simulink model "Motor_Model"  (R2020b)
settings: Solver=VariableStepAuto  StartTime=0.0  StopTime=5  RelTol=1e-3
libraries: fl_lib x114, ee_lib x34, nesl_utility x20
(part 1 of 2)
settings Model: SimulationMode=accelerator  Creator=rubse  LastModifiedBy=rubse

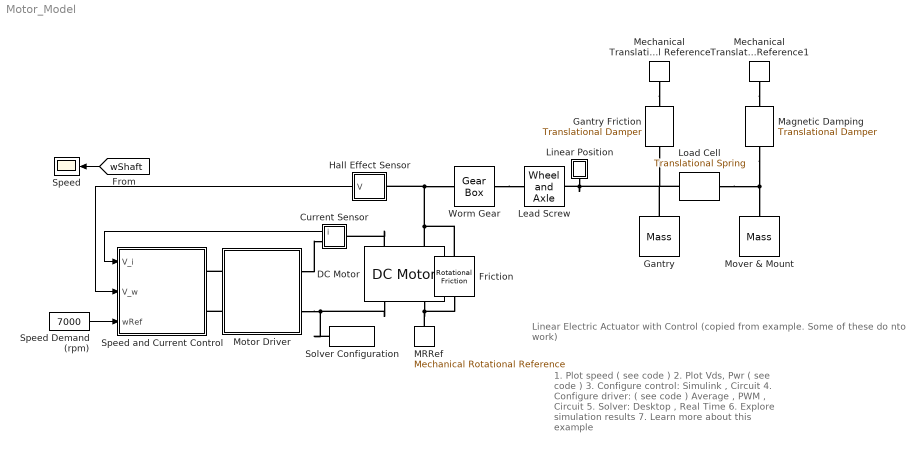
== system Motor_Model ==
  note: Linear Electric Actuator with Control
      | (copied from example. Some of these do nto work)
  note: 1. Plot speed ( see code )
      | 2. Plot Vds, Pwr ( see code )
      | 3. Configure control: Simulink , Circuit
      | 4. Configure driver: ( see code )
      | Average , PWM , Circuit
      | 5. Solver: Desktop , Real Time
      | 6. Explore simulation results
      | 7. Learn more about this example
  Current Sensor : Subsystem
  DC Motor : ee_lib/Electromechanical/Brushed Motors/DC Motor  field_option=ee.enum.field_option.pm  Rf=100 Ohm  Lf=1 H  Laf=0.15 H  If0=0 A  parameterization=ee.enum.dcparam_option.circuit_param  Ra=0.0787 Ohm  La=0.121e-3 H  emf_or_torque=ee.enum.emf_or_torque.ki  Kv=0.0637 V/rpm  Ki=32.3e-3 N*m/A  T_stall=2.4e-4 N*m  w_max=1.91e+4 rpm  w_rated=1.5e+4 rpm  P_rated=0.08 W  V_rated=1.5 V  J=107 g*cm^2  lam_param=ee.enum.lam_param.damping  lam=1e-08 N*m/(rad/s)  i_noload=0 A  V_i_noload=1.5 V  speed0=0 rpm  enable_fault_armature=ee.enum.faults.faultEnable.no  rev_faulted=1 / 3  G_faulted_armature=1e-5 S  fault_trigger_armature=ee.enum.faults.faultTrigger.temporal  t_fault_armature=1 s  max_permissible_current_armature=inf A  t_fail_on_current_armature=1 s  enable_fault_field=ee.enum.faults.faultEnable.no  G_faulted_field=1e-5 S  fault_trigger_field=ee.enum.faults.faultTrigger.temporal  t_fault_field=1 s  max_permissible_current_field=inf A  t_fail_on_current_field=1 s  fault_action=ee.enum.faults.faultAction.none  alpha=3.93e-3 1/K  Tmeas=25 degC  thermal_mass=100 J/K  initial_temperature=25 degC
      settings: SourceProductName=Electrical
  Friction : fl_lib/Mechanical/Rotational Elements/Rotational Friction  brkwy_trq=0.022 N*m  brkwy_vel=0.03347 rad/s  Col_trq=0.022 N*m  visc_coef=0 N*m/(rad/s)  w_specify=off  w_priority=High  w=0 rad/s  w_nominal_specify=off  w_nominal_unit=rad/s  w_nominal_value=1  t_specify=off  t_priority=High  t=0 N*m  t_nominal_specify=off  t_nominal_unit=N*m  t_nominal_value=1
      settings: SourceProductName=Foundation Library
  Gantry : fl_lib/Mechanical/Translational Elements/Mass  mass=5 kg  num_ports=foundation.enum.numPorts2.one  v_specify=off  v_priority=High  v=0 m/s  v_nominal_specify=off  v_nominal_unit=m/s  v_nominal_value=1  f_specify=off  f_priority=None  f=0 N  f_nominal_specify=off  f_nominal_unit=N  f_nominal_value=1
  Gantry Friction : fl_lib/Mechanical/Translational Elements/Translational Damper  D=0.09 N/(m/s)  v_specify=off  v_priority=None  v=0 m/s  v_nominal_specify=off  v_nominal_unit=m/s  v_nominal_value=1  f_specify=off  f_priority=None  f=0 N  f_nominal_specify=off  f_nominal_unit=N  f_nominal_value=1
  Hall Effect Sensor : Subsystem
  Lead Screw : fl_lib/Mechanical/Mechanisms/Wheel and Axle  R=0.05 m  or=1  t_specify=off  t_priority=High  t=0 N*m  t_nominal_specify=off  t_nominal_unit=N*m  t_nominal_value=1  f_specify=off  f_priority=High  f=0 N  f_nominal_specify=off  f_nominal_unit=N  f_nominal_value=1
      settings: SourceProductName=Foundation Library
  Linear Position : Subsystem
      mask Display: disp('S');
  Load Cell : fl_lib/Mechanical/Translational Elements/Translational Spring  spr_rate=670000 N/m  v_specify=off  v_priority=None  v=0 m/s  v_nominal_specify=off  v_nominal_unit=m/s  v_nominal_value=1  f_specify=off  f_priority=None  f=0 N  f_nominal_specify=off  f_nominal_unit=N  f_nominal_value=1  x_specify=off  x_priority=High  x=0 m  x_nominal_specify=off  x_nominal_unit=m  x_nominal_value=1
  MRRef : fl_lib/Mechanical/Rotational Elements/Mechanical Rotational Reference
      settings: SourceProductName=Foundation Library
  Magnetic Damping : fl_lib/Mechanical/Translational Elements/Translational Damper  D=49.05 N/(m/s)  v_specify=off  v_priority=None  v=0 m/s  v_nominal_specify=off  v_nominal_unit=m/s  v_nominal_value=1  f_specify=off  f_priority=None  f=0 N  f_nominal_specify=off  f_nominal_unit=N  f_nominal_value=1
  Mechanical Translational Reference : fl_lib/Mechanical/Translational Elements/Mechanical Translational Reference
  Mechanical Translational Reference1 : fl_lib/Mechanical/Translational Elements/Mechanical Translational Reference
  Motor Driver : Subsystem  Variant=on  VariantControlMode=label  LabelModeActiveChoice=Circuit
      settings: AttributesFormatString=%<ActiveVariant>
      mask Display:
      | if(strcmp(get_param(gcb,'ActiveVariant'),'Circuit'))
      |     temp_imagename = 'ee_motor_linact_control_drive_circuit.jpg';
      | elseif(strcmp(get_param([gcb '/Abstract/Controlled PWM Voltage'],'pwm_or_av'),'1'))
      |     temp_imagename = 'ee_motor_linact_control_drive_abstract_pwm.jpg';
      | else
      |     temp_imagename = 'ee_motor_linact_control_drive_abstract_continuous.jpg';
      | end
      | 
      | image(imread(temp_imagename));
  Mover & Mount : fl_lib/Mechanical/Translational Elements/Mass  mass=2.03 kg  num_ports=foundation.enum.numPorts2.one  v_specify=off  v_priority=High  v=0 m/s  v_nominal_specify=off  v_nominal_unit=m/s  v_nominal_value=1  f_specify=off  f_priority=None  f=0 N  f_nominal_specify=off  f_nominal_unit=N  f_nominal_value=1
  Solver Configuration : nesl_utility/Solver Configuration  PhysicalDomain=network_engine_domain  SubClassName=solver  LeftPortType=input  RightPortType=generic  Tones=[]  Harmonics=[]  SimulateNoise=off  Profile=off  UseLocalSampling=off  EnableSwitchedLinearOptims=on  FrequencyDomain=off  UseCCode=off  RelTol=0.001  AbsTol=1e-06  MinStep=1e-09  ToWorkspace=off  RevertToSquareIcSolve=off  NumHomotopyIterations=100  PhasorMode=off  PhasorModeNumHarmonics=1  DoDC=off  ResidualTolerance=1e-9  UseLocalSolver=off  LocalSolverChoice=NE_BACKWARD_EULER_ADVANCER  LocalSolverSampleTime=0.0001  DoFixedCost=off  MaxNonlinIter=3  MaxModeIter=2  ComputeImpulses=off  ImpulseIterations=2  LinearAlgebra=auto  EquationFormulation=NE_TIME_EF  DelaysMemoryBudget=1024  AutomaticFiltering=on  FilteringTimeConstant=0.001  PartitionStorageMethod=AS_NEEDED  PartitionMemoryBudget=1024  PartitionMethod=FAST
      settings: SourceProductName=Utilities
  Speed : Scope
  Speed Demand (rpm) : Constant  Value=7000
  Speed and Current Control : Subsystem  Variant=on  VariantControlMode=label  LabelModeActiveChoice=Simulink
      settings: AttributesFormatString=%<ActiveVariant>
      mask Display:
      | blk = find_system(gcbh, 'SearchDepth', 1, 'Parent', gcb, 'VariantObject', get_param(gcb,'activevariant'));
      | eval(get_param(blk, 'MaskDisplay'));
  Worm Gear : fl_lib/Mechanical/Mechanisms/Gear Box  ratio=12  t_in_specify=off  t_in_priority=High  t_in=0 N*m  t_in_nominal_specify=off  t_in_nominal_unit=N*m  t_in_nominal_value=1  t_out_specify=off  t_out_priority=High  t_out=0 N*m  t_out_nominal_specify=off  t_out_nominal_unit=N*m  t_out_nominal_value=1
      settings: SourceProductName=Foundation Library
  wires:
  Speed Demand (rpm)/1 -> Speed and Current Control/3(wRef)
  Current Sensor/1(i) -> Speed and Current Control/1(V_i)
  Hall Effect Sensor/1(V) -> Speed and Current Control/2(V_w)
  [wShaft] -> Speed/1
  connections:
  DC Motor/RConn2 -- MRRef/LConn1 -- Friction/RConn1
  DC Motor/LConn2 -- Worm Gear/LConn1 -- Hall Effect Sensor/LConn1 -- Friction/LConn1
  Linear Position/LConn1 -- Load Cell/LConn1 -- Gantry/LConn1 -- Gantry Friction/RConn1 -- Lead Screw/RConn1
  Solver Configuration/RConn1 -- DC Motor/RConn1 -- Motor Driver/RConn2
  Motor Driver/LConn2 -- Speed and Current Control/RConn2
  Motor Driver/LConn1 -- Speed and Current Control/RConn1
  DC Motor/LConn1 -- Current Sensor/LConn1
  Motor Driver/RConn1 -- Current Sensor/RConn1
  Worm Gear/RConn1 -- Lead Screw/LConn1
  Mechanical Translational Reference/LConn1 -- Gantry Friction/LConn1
  Load Cell/RConn1 -- Mover & Mount/LConn1 -- Magnetic Damping/RConn1
  Mechanical Translational Reference1/LConn1 -- Magnetic Damping/LConn1

== system Motor_Model/Current Sensor ==
  2kHz Lowpass Filter : TransferFcn  Denominator=[1/(2*pi*1000) 1]
  Current Sensor : fl_lib/Electrical/Electrical Sensors/Current Sensor
      settings: SourceProductName=Foundation Library
  Motor Current : Scope
  PS-Simulink Converter 2 : nesl_utility/PS-Simulink Converter  PhysicalDomain=network_engine_domain  SubClassName=ps_output  LeftPortType=input  RightPortType=output  PseudoPeriodic=off  Frequencies=[]  Unit=A  AffineConversion=off
      settings: SourceProductName=Utilities
  + : PMIOPort  Side=Right
  - : PMIOPort  Port=2  Side=Left
  i : Outport  VectorParamsAs1DForOutWhenUnconnected=off
  wires:
  PS-Simulink Converter 2/1 -> 2kHz Lowpass Filter/1, Motor Current/1  "Current (A)"
  2kHz Lowpass Filter/1 -> i/1
  connections:
  +/RConn1 -- Current Sensor/LConn1
  -/RConn1 -- Current Sensor/RConn2
  Current Sensor/RConn1 -- PS-Simulink Converter 2/LConn1

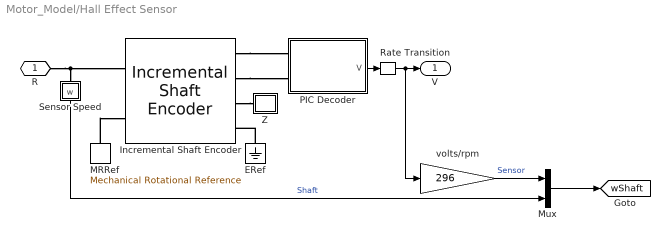
== system Motor_Model/Hall Effect Sensor ==
  ERef : fl_lib/Electrical/Electrical Elements/Electrical Reference
      settings: SourceProductName=Foundation Library
  Incremental Shaft Encoder : ee_lib/Sensors & Transducers/Incremental Shaft Encoder  NPulse=2  Vm=5 V  angle0=-1 deg
      settings: SourceProductName=Electrical  InternalSimscapePortConfiguration="{\"Bottom\":[],\"Left\":[{\"id\":\"R\",\"label\":\"R\",\"type\":\"foundation.mechanical.rotational.rotational\"},{\"id\":\"C\",\"label\":\"C\",\"type\":\"foundation.mechanical.rotational.rotational\"}],\"Right\":[{\"id\":\"A\",\"label\":\"A\",\"type\":\"foundation.electrical.electrical\"},{\"id\":\"B\",\"label\":\"B\",\"type\":\"foundation.electrical.electrical\"},{\"id\":\"Z\",\"label\":\"Z\",\"type\":\"foundation.electrical.electrical\"},{\"id\":\"GND\",\"label\":\"REF\",\"type\":\"foundation.electrical.electrical\"}],\"Top\":[]}"
  MRRef : fl_lib/Mechanical/Rotational Elements/Mechanical Rotational Reference
      settings: SourceProductName=Foundation Library
  Mux : Mux  Inputs=2
  PIC Decoder : Subsystem
  Rate Transition : RateTransition
  Sensor Speed : Subsystem
      mask Display: disp('w')
  Z : Subsystem
  volts/rpm : Gain  Gain=296
  R : PMIOPort  Side=Left
  V : Outport  VectorParamsAs1DForOutWhenUnconnected=off
  tag scope: wShaft=global
  wires:
  PIC Decoder/1(V) -> Rate Transition/1
  Rate Transition/1 -> V/1, volts/rpm/1
  Mux/1 -> [wShaft]
  volts/rpm/1 -> Mux/1  "Sensor"
  Sensor Speed/1(w) -> Mux/2  "Shaft"
  connections:
  MRRef/LConn1 -- Incremental Shaft Encoder/LConn2
  R/RConn1 -- Incremental Shaft Encoder/LConn1 -- Sensor Speed/LConn1
  ERef/LConn1 -- Incremental Shaft Encoder/RConn4
  Incremental Shaft Encoder/RConn3 -- Z/LConn1
  Incremental Shaft Encoder/RConn1 -- PIC Decoder/LConn1
  Incremental Shaft Encoder/RConn2 -- PIC Decoder/LConn2

== system Motor_Model/Linear Position ==
  Linear Position (mm) : Scope
  Linear Speed (mm/s) : Scope
  MTRef : fl_lib/Mechanical/Translational Elements/Mechanical Translational Reference
      settings: SourceProductName=Foundation Library
  Motion Sensor : fl_lib/Mechanical/Mechanical Sensors/Ideal Translational Motion Sensor  offset=0 m
      settings: SourceProductName=Foundation Library
  PS-Simulink Converter 1 : nesl_utility/PS-Simulink Converter  PhysicalDomain=network_engine_domain  SubClassName=ps_output  LeftPortType=input  RightPortType=output  PseudoPeriodic=off  Frequencies=[]  Unit=mm/s  AffineConversion=off
      settings: SourceProductName=Utilities
  PS-Simulink Converter 3 : nesl_utility/PS-Simulink Converter  PhysicalDomain=network_engine_domain  SubClassName=ps_output  LeftPortType=input  RightPortType=output  PseudoPeriodic=off  Frequencies=[]  Unit=mm  AffineConversion=off
      settings: SourceProductName=Utilities
  P : PMIOPort  Side=Left
  wires:
  PS-Simulink Converter 3/1 -> Linear Position (mm)/1
  PS-Simulink Converter 1/1 -> Linear Speed (mm/s)/1
  connections:
  Motion Sensor/RConn1 -- MTRef/LConn1
  Motion Sensor/RConn3 -- PS-Simulink Converter 3/LConn1
  P/RConn1 -- Motion Sensor/LConn1
  Motion Sensor/RConn2 -- PS-Simulink Converter 1/LConn1

== system Motor_Model/Motor Driver ==
  Abstract : Subsystem  Tag=PublishSubsystem  VariantControl=Abstract
  Circuit : Subsystem  Tag=PublishSubsystem  VariantControl=Circuit
  + : PMIOPort  Side=Right
  - : PMIOPort  Port=2  Side=Right
  +ref : PMIOPort  Port=3  Side=Left
  REV : PMIOPort  Port=4  Side=Left

== system Motor_Model/Speed and Current Control ==
  V_i : Inport
  V_w : Inport  Port=2
  wRef : Inport  Port=3
  Circuit : Subsystem  VariantControl=Circuit
      mask Display: image(imread('ee_motor_linact_control_ctrl_circuit.jpg'));
  Simulink : Subsystem  VariantControl=Simulink
      mask Display: image('ee_motor_linact_control_ctrl_simulink.jpg');
  Vr : PMIOPort  Side=Right
  REV : PMIOPort  Port=2  Side=Right

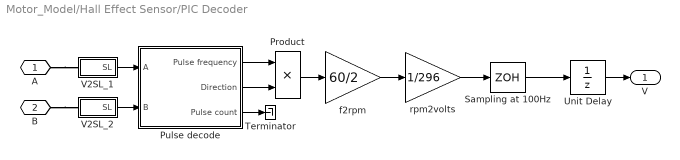
== system Motor_Model/Hall Effect Sensor/PIC Decoder ==
  Product : Product  RndMeth=Zero
  Pulse decode : Subsystem
  Sampling at 100Hz : ZeroOrderHold  SampleTime=0.01
  Terminator : Terminator
  Unit Delay : UnitDelay  SampleTime=0.01  HasFrameUpgradeWarning=on
  V2SL_1 : Subsystem
  V2SL_2 : Subsystem
  f2rpm : Gain  Gain=60/2
  rpm2volts : Gain  Gain=1/296
  A : PMIOPort  Side=Left
  B : PMIOPort  Port=2  Side=Left
  V : Outport  VectorParamsAs1DForOutWhenUnconnected=off
  wires:
  Product/1 -> f2rpm/1
  Pulse decode/2(Direction) -> Product/2
  Pulse decode/1(Pulse frequency) -> Product/1
  Pulse decode/3(Pulse count) -> Terminator/1
  f2rpm/1 -> rpm2volts/1
  rpm2volts/1 -> Sampling at 100Hz/1
  V2SL_1/1(SL) -> Pulse decode/1(A)
  V2SL_2/1(SL) -> Pulse decode/2(B)
  Sampling at 100Hz/1 -> Unit Delay/1
  Unit Delay/1 -> V/1
  connections:
  A/RConn1 -- V2SL_1/LConn1
  B/RConn1 -- V2SL_2/LConn1

== system Motor_Model/Hall Effect Sensor/Sensor Speed ==
  MRRef5 : fl_lib/Mechanical/Rotational Elements/Mechanical Rotational Reference
      settings: SourceProductName=Foundation Library
  Motion Sensor : fl_lib/Mechanical/Mechanical Sensors/Ideal Rotational Motion Sensor  wrap_angle=simscape.enum.onoff.off  offset=0 rad
      settings: SourceProductName=Foundation Library
  PS-Simulink Converter 2 : nesl_utility/PS-Simulink Converter  PhysicalDomain=network_engine_domain  SubClassName=ps_output  LeftPortType=input  RightPortType=output  PseudoPeriodic=off  Frequencies=[]  Unit=rpm  AffineConversion=off
      settings: SourceProductName=Utilities
  R : PMIOPort  Side=Left
  w : Outport  VectorParamsAs1DForOutWhenUnconnected=off
  wires:
  PS-Simulink Converter 2/1 -> w/1
  connections:
  Motion Sensor/RConn2 -- PS-Simulink Converter 2/LConn1
  R/RConn1 -- Motion Sensor/LConn1
  MRRef5/LConn1 -- Motion Sensor/RConn1

== system Motor_Model/Hall Effect Sensor/Z ==
  ERef : fl_lib/Electrical/Electrical Elements/Electrical Reference
      settings: SourceProductName=Foundation Library
  PS-Simulink Converter 2 : nesl_utility/PS-Simulink Converter  PhysicalDomain=network_engine_domain  SubClassName=ps_output  LeftPortType=input  RightPortType=output  PseudoPeriodic=off  Frequencies=[]  Unit=V  AffineConversion=off
      settings: SourceProductName=Utilities
  Voltage Sensor : fl_lib/Electrical/Electrical Sensors/Voltage Sensor
      settings: SourceProductName=Foundation Library
  Vz : Scope
  u : PMIOPort  Side=Left
  wires:
  PS-Simulink Converter 2/1 -> Vz/1
  connections:
  Voltage Sensor/RConn2 -- ERef/LConn1
  Voltage Sensor/RConn1 -- PS-Simulink Converter 2/LConn1
  u/RConn1 -- Voltage Sensor/LConn1

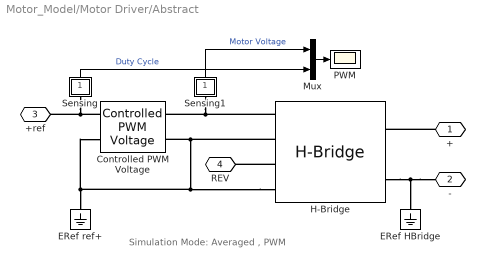
== system Motor_Model/Motor Driver/Abstract ==
  note: Simulation Mode: Averaged , PWM
  Controlled PWM Voltage : ee_lib/Integrated Circuits/Controlled PWM Voltage  F=10000 Hz  TD=0 s  pulse_width_offset=0 s  pulse_min=0 s  Vmin=0 V  Vmax=5 V  Vm=5 V  pwm_or_av=2  event_type=1  sample_time=1e-6 s  u_min=0  u_max=1
      settings: SourceProductName=Electrical
  ERef HBridge : fl_lib/Electrical/Electrical Elements/Electrical Reference
      settings: SourceProductName=Foundation Library
  ERef ref+ : fl_lib/Electrical/Electrical Elements/Electrical Reference
      settings: SourceProductName=Foundation Library
  H-Bridge : ee_lib/Semiconductors & Converters/Converters/H-Bridge  supply_ports=ee.enum.supply_ports.hidesupply  Venable=2.5 V  Vmax=5 V  Vreverse=2.5 V  Vbrake=2.5 V  Vm=24 V  pwm_or_av=2  regenerative_braking_mode=2  discontinuous=0  freewheeling_mode=1  Ron=0.1 Ohm  Don=0.1 Ohm  Goff=1e-6 S  Rload=10 Ohm  Lload=1e-5 H  F=10 kHz  thermal_mass=100 J/K  initial_temperature=298.15 K  Ron2=0.1 Ohm  Don2=0.05 Ohm  Tmeas=298.15 K  Tmeas2=398.15 K
      settings: SourceProductName=Electrical
  Mux : Mux  Inputs=2
  PWM : Scope
  Sensing : Subsystem
      mask Display: disp('V')
  Sensing1 : Subsystem
      mask Display: disp('V')
  + : PMIOPort  Side=Right
  - : PMIOPort  Port=2  Side=Right
  +ref : PMIOPort  Port=3  Side=Left
  REV : PMIOPort  Port=4  Side=Left
  wires:
  Mux/1 -> PWM/1
  Sensing/1(Out1) -> Mux/2  "Duty Cycle"
  Sensing1/1(Out1) -> Mux/1  "Motor Voltage"
  connections:
  H-Bridge/LConn3 -- REV/RConn1
  Controlled PWM Voltage/LConn1 -- Sensing/LConn1 -- +ref/RConn1
  H-Bridge/LConn4 -- Controlled PWM Voltage/RConn2 -- H-Bridge/LConn2 -- Controlled PWM Voltage/LConn2 -- ERef ref+/LConn1
  H-Bridge/LConn1 -- Sensing1/LConn1 -- Controlled PWM Voltage/RConn1
  -/RConn1 -- ERef HBridge/LConn1 -- H-Bridge/RConn2
  +/RConn1 -- H-Bridge/RConn1

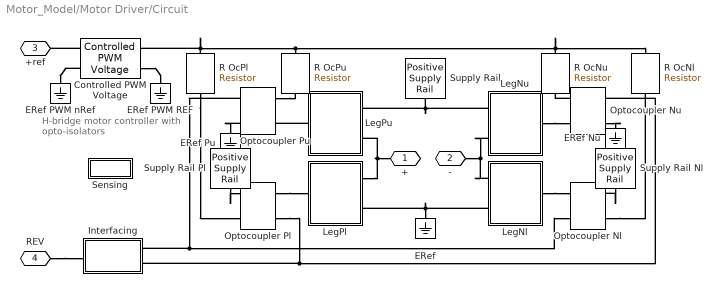
== system Motor_Model/Motor Driver/Circuit ==
  note: H-bridge motor controller
      | with opto-isolators
  Controlled PWM Voltage : ee_lib/Integrated Circuits/Controlled PWM Voltage  F=10000 Hz  TD=0 s  pulse_width_offset=0 s  pulse_min=0 s  Vmin=0 V  Vmax=5 V  Vm=5 V  pwm_or_av=1  event_type=1  sample_time=1e-6 s  u_min=0  u_max=1
      settings: SourceProductName=Electrical
  ERef : fl_lib/Electrical/Electrical Elements/Electrical Reference
      settings: SourceProductName=Foundation Library
  ERef PWM REF : fl_lib/Electrical/Electrical Elements/Electrical Reference
      settings: SourceProductName=Foundation Library
  ERef PWM nRef : fl_lib/Electrical/Electrical Elements/Electrical Reference
      settings: SourceProductName=Foundation Library
  ERef Nu : fl_lib/Electrical/Electrical Elements/Electrical Reference
      settings: SourceProductName=Foundation Library
  ERef Pu : fl_lib/Electrical/Electrical Elements/Electrical Reference
      settings: SourceProductName=Foundation Library
  Interfacing : Subsystem
  LegNl : Subsystem
      mask Display:
      | patch([96+30;0-30;0-30;96+30], [0+10;0+10;227-10;227-10], [1;1;1])
      | plot([96.6109160799533;96.4198282107139;95.8484048836359;94.9021492177306;93.5901741723367;91.9251147843401;89.9230064858609;87.6031306742773;84.9878290218281;82.1022883130956;78.9742978825019;75.6339819878271;72.1135096971394;68.4467850830839;64.6691207081296;60.8168975452888;56.927214609459;53.0375316736292;49.1853085107884;45.4076441358342;41.7409195217787;38.220447231091;34.8801313364162;31.7521409058224;28.86660019709;26.2512985446407;23.9314227330572;21.929314434578;20.2642550465813;18.9522800011875;18.0060243352822;17.4346010082041;17.2435131389648;17.4346010082041;18.0060243352822;18.9522800011875;20.2642550465814;21.9293144345781;23.9314227330573;26.2512985446408;28.8666001970901;31.7521409058226;34.8801313364163;38.2204472310911;41.7409195217788;45.4076441358342;49.1853085107884;53.0375316736292;56.927214609459;60.8168975452889;64.6691207081297;68.4467850830839;72.1135096971393;75.633981987827;78.9742978825018;82.1022883130955;84.9878290218281;87.6031306742773;89.9230064858608;91.9251147843399;93.5901741723367;94.9021492177305;95.8484048836358;96.4198282107139;96.6109160799533;96.6109160799533], [113.618216710165;109.728533774335;105.876310611494;102.09864623654;98.4319216224848;94.9114493317971;91.5711334371223;88.4431430065286;85.5576022977961;82.9423006453468;80.6224248337633;78.6203165352841;76.9552571472875;75.6432821018936;74.6970264359883;74.1256031089102;73.9345152396709;74.1256031089102;74.6970264359883;75.6432821018936;76.9552571472875;78.6203165352842;80.6224248337634;82.9423006453469;85.5576022977961;88.4431430065287;91.5711334371223;94.9114493317971;98.4319216224849;102.09864623654;105.876310611495;109.728533774335;113.618216710165;117.507899645995;121.360122808836;125.13778718379;128.804511797846;132.324984088533;135.665299983208;138.793290413802;141.678831122534;144.294132774983;146.614008586567;148.616116885046;150.281176273043;151.593151318437;152.539406984342;153.11083031142;153.301918180659;153.11083031142;152.539406984342;151.593151318437;150.281176273043;148.616116885046;146.614008586567;144.294132774983;141.678831122534;138.793290413802;135.665299983208;132.324984088533;128.804511797846;125.13778718379;121.360122808836;117.507899645995;113.618216710165;113.618216710165])
      | plot([33.9988537598401;34.5027737785131], [113.618216710165;113.618216710165])
      | plot([0.236212508752942;34.2508137691766], [113.618216710165;113.618216710165])
      | plot([34.2508137691766;34.2508137691766], [136.294617550448;90.9418158698827])
      | plot([45.5890141893178;45.5890141893178], [136.294617550448;90.9418158698827])
      | plot([45.5890141893178;68.2654150296003], [130.625517340377;130.625517340377])
      | plot([68.2654150296003;68.2654150296003], [130.625517340377;170.309218810871])
      | plot([68.2654150296003;93.776365974918], [170.309218810871;170.309218810871])
      | plot([45.5890141893178;68.2654150296003], [96.6109160799533;96.6109160799533])
      | plot([68.2654150296003;68.2654150296003], [96.6109160799533;56.927214609459])
      | plot([68.2654150296003;96.6109160799533], [56.927214609459;56.927214609459])
      | plot([45.5890141893178;68.2654150296003], [113.618216710165;113.618216710165])
      | plot([68.2654150296003;68.2654150296003], [130.618216710165;113.6109160799533])
      | plot([62.2581143993884;51.5963148195297;62.2581143993884], [124.956417130306;113.618216710165;102.280016290024])
  LegNu : Subsystem
      mask Display:
      | patch([96+30;0-30;0-30;96+30], [0+10;0+10;227-10;227-10], [1;1;1])
      | plot([96.6109160799533;96.4198282107139;95.8484048836359;94.9021492177306;93.5901741723367;91.9251147843401;89.9230064858609;87.6031306742773;84.9878290218281;82.1022883130956;78.9742978825019;75.6339819878271;72.1135096971394;68.4467850830839;64.6691207081296;60.8168975452888;56.927214609459;53.0375316736292;49.1853085107884;45.4076441358342;41.7409195217787;38.220447231091;34.8801313364162;31.7521409058224;28.86660019709;26.2512985446407;23.9314227330572;21.929314434578;20.2642550465813;18.9522800011875;18.0060243352822;17.4346010082041;17.2435131389648;17.4346010082041;18.0060243352822;18.9522800011875;20.2642550465814;21.9293144345781;23.9314227330573;26.2512985446408;28.8666001970901;31.7521409058226;34.8801313364163;38.2204472310911;41.7409195217788;45.4076441358342;49.1853085107884;53.0375316736292;56.927214609459;60.8168975452889;64.6691207081297;68.4467850830839;72.1135096971393;75.633981987827;78.9742978825018;82.1022883130955;84.9878290218281;87.6031306742773;89.9230064858608;91.9251147843399;93.5901741723367;94.9021492177305;95.8484048836358;96.4198282107139;96.6109160799533;96.6109160799533], [113.618216710165;109.728533774335;105.876310611494;102.09864623654;98.4319216224848;94.9114493317971;91.5711334371223;88.4431430065286;85.5576022977961;82.9423006453468;80.6224248337633;78.6203165352841;76.9552571472875;75.6432821018936;74.6970264359883;74.1256031089102;73.9345152396709;74.1256031089102;74.6970264359883;75.6432821018936;76.9552571472875;78.6203165352842;80.6224248337634;82.9423006453469;85.5576022977961;88.4431430065287;91.5711334371223;94.9114493317971;98.4319216224849;102.09864623654;105.876310611495;109.728533774335;113.618216710165;117.507899645995;121.360122808836;125.13778718379;128.804511797846;132.324984088533;135.665299983208;138.793290413802;141.678831122534;144.294132774983;146.614008586567;148.616116885046;150.281176273043;151.593151318437;152.539406984342;153.11083031142;153.301918180659;153.11083031142;152.539406984342;151.593151318437;150.281176273043;148.616116885046;146.614008586567;144.294132774983;141.678831122534;138.793290413802;135.665299983208;132.324984088533;128.804511797846;125.13778718379;121.360122808836;117.507899645995;113.618216710165;113.618216710165])
      | plot([33.9988537598401;34.5027737785131], [113.618216710165;113.618216710165])
      | plot([0.236212508752942;34.2508137691766], [113.618216710165;113.618216710165])
      | plot([34.2508137691766;34.2508137691766], [136.294617550448;90.9418158698827])
      | plot([45.5890141893178;45.5890141893178], [136.294617550448;90.9418158698827])
      | plot([45.5890141893178;68.2654150296003], [130.625517340377;130.625517340377])
      | plot([68.2654150296003;68.2654150296003], [130.625517340377;170.309218810871])
      | plot([68.2654150296003;93.776365974918], [170.309218810871;170.309218810871])
      | plot([45.5890141893178;68.2654150296003], [96.6109160799533;96.6109160799533])
      | plot([68.2654150296003;68.2654150296003], [96.6109160799533;56.927214609459])
      | plot([68.2654150296003;96.6109160799533], [56.927214609459;56.927214609459])
      | plot([45.5890141893178;68.2654150296003], [113.618216710165;113.618216710165])
      | plot([68.2654150296003;68.2654150296003], [130.618216710165;113.6109160799533])
      | plot([51.5963148195297;62.2581143993884;51.5963148195297], [124.956417130306;113.618216710165;102.280016290024])
  LegPl : Subsystem
      mask Display:
      | patch([96+30;0-30;0-30;96+30], [0+10;0+10;227-10;227-10], [1;1;1])
      | plot([96.6109160799533;96.4198282107139;95.8484048836359;94.9021492177306;93.5901741723367;91.9251147843401;89.9230064858609;87.6031306742773;84.9878290218281;82.1022883130956;78.9742978825019;75.6339819878271;72.1135096971394;68.4467850830839;64.6691207081296;60.8168975452888;56.927214609459;53.0375316736292;49.1853085107884;45.4076441358342;41.7409195217787;38.220447231091;34.8801313364162;31.7521409058224;28.86660019709;26.2512985446407;23.9314227330572;21.929314434578;20.2642550465813;18.9522800011875;18.0060243352822;17.4346010082041;17.2435131389648;17.4346010082041;18.0060243352822;18.9522800011875;20.2642550465814;21.9293144345781;23.9314227330573;26.2512985446408;28.8666001970901;31.7521409058226;34.8801313364163;38.2204472310911;41.7409195217788;45.4076441358342;49.1853085107884;53.0375316736292;56.927214609459;60.8168975452889;64.6691207081297;68.4467850830839;72.1135096971393;75.633981987827;78.9742978825018;82.1022883130955;84.9878290218281;87.6031306742773;89.9230064858608;91.9251147843399;93.5901741723367;94.9021492177305;95.8484048836358;96.4198282107139;96.6109160799533;96.6109160799533], [113.618216710165;109.728533774335;105.876310611494;102.09864623654;98.4319216224848;94.9114493317971;91.5711334371223;88.4431430065286;85.5576022977961;82.9423006453468;80.6224248337633;78.6203165352841;76.9552571472875;75.6432821018936;74.6970264359883;74.1256031089102;73.9345152396709;74.1256031089102;74.6970264359883;75.6432821018936;76.9552571472875;78.6203165352842;80.6224248337634;82.9423006453469;85.5576022977961;88.4431430065287;91.5711334371223;94.9114493317971;98.4319216224849;102.09864623654;105.876310611495;109.728533774335;113.618216710165;117.507899645995;121.360122808836;125.13778718379;128.804511797846;132.324984088533;135.665299983208;138.793290413802;141.678831122534;144.294132774983;146.614008586567;148.616116885046;150.281176273043;151.593151318437;152.539406984342;153.11083031142;153.301918180659;153.11083031142;152.539406984342;151.593151318437;150.281176273043;148.616116885046;146.614008586567;144.294132774983;141.678831122534;138.793290413802;135.665299983208;132.324984088533;128.804511797846;125.13778718379;121.360122808836;117.507899645995;113.618216710165;113.618216710165])
      | plot([33.9988537598401;34.5027737785131], [113.618216710165;113.618216710165])
      | plot([0.236212508752942;34.2508137691766], [113.618216710165;113.618216710165])
      | plot([34.2508137691766;34.2508137691766], [136.294617550448;90.9418158698827])
      | plot([45.5890141893178;45.5890141893178], [136.294617550448;90.9418158698827])
      | plot([45.5890141893178;68.2654150296003], [130.625517340377;130.625517340377])
      | plot([68.2654150296003;68.2654150296003], [130.625517340377;170.309218810871])
      | plot([68.2654150296003;93.776365974918], [170.309218810871;170.309218810871])
      | plot([45.5890141893178;68.2654150296003], [96.6109160799533;96.6109160799533])
      | plot([68.2654150296003;68.2654150296003], [96.6109160799533;56.927214609459])
      | plot([68.2654150296003;96.6109160799533], [56.927214609459;56.927214609459])
      | plot([45.5890141893178;68.2654150296003], [113.618216710165;113.618216710165])
      | plot([68.2654150296003;68.2654150296003], [130.618216710165;113.6109160799533])
      | plot([62.2581143993884;51.5963148195297;62.2581143993884], [124.956417130306;113.618216710165;102.280016290024])
  LegPu : Subsystem  Tag=PublishSubsystem
      mask Display:
      | patch([96+30;0-30;0-30;96+30], [0+10;0+10;227-10;227-10], [1;1;1])
      | plot([96.6109160799533;96.4198282107139;95.8484048836359;94.9021492177306;93.5901741723367;91.9251147843401;89.9230064858609;87.6031306742773;84.9878290218281;82.1022883130956;78.9742978825019;75.6339819878271;72.1135096971394;68.4467850830839;64.6691207081296;60.8168975452888;56.927214609459;53.0375316736292;49.1853085107884;45.4076441358342;41.7409195217787;38.220447231091;34.8801313364162;31.7521409058224;28.86660019709;26.2512985446407;23.9314227330572;21.929314434578;20.2642550465813;18.9522800011875;18.0060243352822;17.4346010082041;17.2435131389648;17.4346010082041;18.0060243352822;18.9522800011875;20.2642550465814;21.9293144345781;23.9314227330573;26.2512985446408;28.8666001970901;31.7521409058226;34.8801313364163;38.2204472310911;41.7409195217788;45.4076441358342;49.1853085107884;53.0375316736292;56.927214609459;60.8168975452889;64.6691207081297;68.4467850830839;72.1135096971393;75.633981987827;78.9742978825018;82.1022883130955;84.9878290218281;87.6031306742773;89.9230064858608;91.9251147843399;93.5901741723367;94.9021492177305;95.8484048836358;96.4198282107139;96.6109160799533;96.6109160799533], [113.618216710165;109.728533774335;105.876310611494;102.09864623654;98.4319216224848;94.9114493317971;91.5711334371223;88.4431430065286;85.5576022977961;82.9423006453468;80.6224248337633;78.6203165352841;76.9552571472875;75.6432821018936;74.6970264359883;74.1256031089102;73.9345152396709;74.1256031089102;74.6970264359883;75.6432821018936;76.9552571472875;78.6203165352842;80.6224248337634;82.9423006453469;85.5576022977961;88.4431430065287;91.5711334371223;94.9114493317971;98.4319216224849;102.09864623654;105.876310611495;109.728533774335;113.618216710165;117.507899645995;121.360122808836;125.13778718379;128.804511797846;132.324984088533;135.665299983208;138.793290413802;141.678831122534;144.294132774983;146.614008586567;148.616116885046;150.281176273043;151.593151318437;152.539406984342;153.11083031142;153.301918180659;153.11083031142;152.539406984342;151.593151318437;150.281176273043;148.616116885046;146.614008586567;144.294132774983;141.678831122534;138.793290413802;135.665299983208;132.324984088533;128.804511797846;125.13778718379;121.360122808836;117.507899645995;113.618216710165;113.618216710165])
      | plot([33.9988537598401;34.5027737785131], [113.618216710165;113.618216710165])
      | plot([0.236212508752942;34.2508137691766], [113.618216710165;113.618216710165])
      | plot([34.2508137691766;34.2508137691766], [136.294617550448;90.9418158698827])
      | plot([45.5890141893178;45.5890141893178], [136.294617550448;90.9418158698827])
      | plot([45.5890141893178;68.2654150296003], [130.625517340377;130.625517340377])
      | plot([68.2654150296003;68.2654150296003], [130.625517340377;170.309218810871])
      | plot([68.2654150296003;93.776365974918], [170.309218810871;170.309218810871])
      | plot([45.5890141893178;68.2654150296003], [96.6109160799533;96.6109160799533])
      | plot([68.2654150296003;68.2654150296003], [96.6109160799533;56.927214609459])
      | plot([68.2654150296003;96.6109160799533], [56.927214609459;56.927214609459])
      | plot([45.5890141893178;68.2654150296003], [113.618216710165;113.618216710165])
      | plot([68.2654150296003;68.2654150296003], [130.618216710165;113.6109160799533])
      | plot([51.5963148195297;62.2581143993884;51.5963148195297], [124.956417130306;113.618216710165;102.280016290024])
  Optocoupler Nl : ee_lib/Semiconductors & Converters/Optocoupler  CTR=0.2  prmExp=1  I12="[  0.001 0.015 ] A"  V12="[  0.9 1.05 ] V"  IS=1e-10 A  ec=2  RS=0 Ohm  Tmeas=298.15 K  C_param=1  CJ=50 pF  CJ0=50 pF  VJ=1 V  Mgrad=0.5  Vvec="[  0.1 10 100 ] V"  Cvec="[  3.5 1 0.4 ] pF"  FC=0.5  T_param=1  IS_T2=1.8e-8 A  I1_T2=0.029 A  V1_T2=1.05 V  Tmeas2=125 degC  EG_param=1  EG=1.11 eV  XTI_param=1  XTI=3  Tdevice=25 degC  i_capacitor_specify=off  i_capacitor_priority=High  i_capacitor=0 A  i_capacitor_nominal_specify=off  i_capacitor_nominal_unit=A  i_capacitor_nominal_value=1  v_capacitor_specify=off  v_capacitor_priority=None  v_capacitor=0 V  v_capacitor_nominal_specify=off  v_capacitor_nominal_unit=V  v_capacitor_nominal_value=1  thermal_network_parameterization=ee.enum.thermalNetworkTopology.cauer  Rth=[0, 10] K/W  Rth_Foster=[4, 6] K/W  thermal_mass_parameterization=ee.enum.thermalNetwork.timeconstant  thermal_mass=[0, 1] J/K  thermal_mass_Foster=[1.5, 3] J/K  thermal_time_constant=[0, 10] s  thermal_time_constant_Foster=[6, 18] s  thermal_mass_initial_temperatures=[25, 25] degC
      settings: SourceProductName=Electrical  InternalSimscapePortConfiguration="{\"Bottom\":[],\"Left\":[{\"id\":\"p\",\"label\":\"\",\"type\":\"foundation.electrical.electrical\"},{\"id\":\"C\",\"label\":\"\",\"type\":\"foundation.electrical.electrical\"}],\"Right\":[{\"id\":\"n\",\"label\":\"\",\"type\":\"foundation.electrical.electrical\"},{\"id\":\"E\",\"label\":\"\",\"type\":\"foundation.electrical.electrical\"}],\"Top\":[]}"
  Optocoupler Nu : ee_lib/Semiconductors & Converters/Optocoupler  CTR=0.2  prmExp=1  I12="[  0.001 0.015 ] A"  V12="[  0.9 1.05 ] V"  IS=1e-10 A  ec=2  RS=0 Ohm  Tmeas=298.15 K  C_param=1  CJ=50 pF  CJ0=50 pF  VJ=1 V  Mgrad=0.5  Vvec="[  0.1 10 100 ] V"  Cvec="[  3.5 1 0.4 ] pF"  FC=0.5  T_param=1  IS_T2=1.8e-8 A  I1_T2=0.029 A  V1_T2=1.05 V  Tmeas2=125 degC  EG_param=1  EG=1.11 eV  XTI_param=1  XTI=3  Tdevice=25 degC  i_capacitor_specify=off  i_capacitor_priority=High  i_capacitor=0 A  i_capacitor_nominal_specify=off  i_capacitor_nominal_unit=A  i_capacitor_nominal_value=1  v_capacitor_specify=off  v_capacitor_priority=None  v_capacitor=0 V  v_capacitor_nominal_specify=off  v_capacitor_nominal_unit=V  v_capacitor_nominal_value=1  thermal_network_parameterization=ee.enum.thermalNetworkTopology.cauer  Rth=[0, 10] K/W  Rth_Foster=[4, 6] K/W  thermal_mass_parameterization=ee.enum.thermalNetwork.timeconstant  thermal_mass=[0, 1] J/K  thermal_mass_Foster=[1.5, 3] J/K  thermal_time_constant=[0, 10] s  thermal_time_constant_Foster=[6, 18] s  thermal_mass_initial_temperatures=[25, 25] degC
      settings: SourceProductName=Electrical  InternalSimscapePortConfiguration="{\"Bottom\":[],\"Left\":[{\"id\":\"p\",\"label\":\"\",\"type\":\"foundation.electrical.electrical\"},{\"id\":\"C\",\"label\":\"\",\"type\":\"foundation.electrical.electrical\"}],\"Right\":[{\"id\":\"n\",\"label\":\"\",\"type\":\"foundation.electrical.electrical\"},{\"id\":\"E\",\"label\":\"\",\"type\":\"foundation.electrical.electrical\"}],\"Top\":[]}"
  Optocoupler Pl : ee_lib/Semiconductors & Converters/Optocoupler  CTR=0.2  prmExp=1  I12="[  0.001 0.015 ] A"  V12="[  0.9 1.05 ] V"  IS=1e-10 A  ec=2  RS=0 Ohm  Tmeas=298.15 K  C_param=1  CJ=50 pF  CJ0=50 pF  VJ=1 V  Mgrad=0.5  Vvec="[  0.1 10 100 ] V"  Cvec="[  3.5 1 0.4 ] pF"  FC=0.5  T_param=1  IS_T2=1.8e-8 A  I1_T2=0.029 A  V1_T2=1.05 V  Tmeas2=125 degC  EG_param=1  EG=1.11 eV  XTI_param=1  XTI=3  Tdevice=25 degC  i_capacitor_specify=off  i_capacitor_priority=High  i_capacitor=0 A  i_capacitor_nominal_specify=off  i_capacitor_nominal_unit=A  i_capacitor_nominal_value=1  v_capacitor_specify=off  v_capacitor_priority=None  v_capacitor=0 V  v_capacitor_nominal_specify=off  v_capacitor_nominal_unit=V  v_capacitor_nominal_value=1  thermal_network_parameterization=ee.enum.thermalNetworkTopology.cauer  Rth=[0, 10] K/W  Rth_Foster=[4, 6] K/W  thermal_mass_parameterization=ee.enum.thermalNetwork.timeconstant  thermal_mass=[0, 1] J/K  thermal_mass_Foster=[1.5, 3] J/K  thermal_time_constant=[0, 10] s  thermal_time_constant_Foster=[6, 18] s  thermal_mass_initial_temperatures=[25, 25] degC
      settings: SourceProductName=Electrical  InternalSimscapePortConfiguration="{\"Bottom\":[],\"Left\":[{\"id\":\"p\",\"label\":\"\",\"type\":\"foundation.electrical.electrical\"},{\"id\":\"C\",\"label\":\"\",\"type\":\"foundation.electrical.electrical\"}],\"Right\":[{\"id\":\"n\",\"label\":\"\",\"type\":\"foundation.electrical.electrical\"},{\"id\":\"E\",\"label\":\"\",\"type\":\"foundation.electrical.electrical\"}],\"Top\":[]}"
  Optocoupler Pu : ee_lib/Semiconductors & Converters/Optocoupler  CTR=0.2  prmExp=1  I12="[  0.001 0.015 ] A"  V12="[  0.9 1.05 ] V"  IS=1e-10 A  ec=2  RS=0 Ohm  Tmeas=298.15 K  C_param=1  CJ=50 pF  CJ0=50 pF  VJ=1 V  Mgrad=0.5  Vvec="[  0.1 10 100 ] V"  Cvec="[  3.5 1 0.4 ] pF"  FC=0.5  T_param=1  IS_T2=1.8e-8 A  I1_T2=0.029 A  V1_T2=1.05 V  Tmeas2=125 degC  EG_param=1  EG=1.11 eV  XTI_param=1  XTI=3  Tdevice=25 degC  i_capacitor_specify=off  i_capacitor_priority=High  i_capacitor=0 A  i_capacitor_nominal_specify=off  i_capacitor_nominal_unit=A  i_capacitor_nominal_value=1  v_capacitor_specify=off  v_capacitor_priority=None  v_capacitor=0 V  v_capacitor_nominal_specify=off  v_capacitor_nominal_unit=V  v_capacitor_nominal_value=1  thermal_network_parameterization=ee.enum.thermalNetworkTopology.cauer  Rth=[0, 10] K/W  Rth_Foster=[4, 6] K/W  thermal_mass_parameterization=ee.enum.thermalNetwork.timeconstant  thermal_mass=[0, 1] J/K  thermal_mass_Foster=[1.5, 3] J/K  thermal_time_constant=[0, 10] s  thermal_time_constant_Foster=[6, 18] s  thermal_mass_initial_temperatures=[25, 25] degC
      settings: SourceProductName=Electrical  InternalSimscapePortConfiguration="{\"Bottom\":[],\"Left\":[{\"id\":\"p\",\"label\":\"\",\"type\":\"foundation.electrical.electrical\"},{\"id\":\"C\",\"label\":\"\",\"type\":\"foundation.electrical.electrical\"}],\"Right\":[{\"id\":\"n\",\"label\":\"\",\"type\":\"foundation.electrical.electrical\"},{\"id\":\"E\",\"label\":\"\",\"type\":\"foundation.electrical.electrical\"}],\"Top\":[]}"
  R OcNl : fl_lib/Electrical/Electrical Elements/Resistor  R=470 Ohm  i_specify=off  i_priority=High  i=0 A  i_nominal_specify=off  i_nominal_unit=A  i_nominal_value=1  v_specify=off  v_priority=High  v=0 V  v_nominal_specify=off  v_nominal_unit=V  v_nominal_value=1
      settings: SourceProductName=Foundation Library
  R OcNu : fl_lib/Electrical/Electrical Elements/Resistor  R=470 Ohm  i_specify=off  i_priority=High  i=0 A  i_nominal_specify=off  i_nominal_unit=A  i_nominal_value=1  v_specify=off  v_priority=High  v=0 V  v_nominal_specify=off  v_nominal_unit=V  v_nominal_value=1
      settings: SourceProductName=Foundation Library
  R OcPl : fl_lib/Electrical/Electrical Elements/Resistor  R=470 Ohm  i_specify=off  i_priority=High  i=0 A  i_nominal_specify=off  i_nominal_unit=A  i_nominal_value=1  v_specify=off  v_priority=High  v=0 V  v_nominal_specify=off  v_nominal_unit=V  v_nominal_value=1
      settings: SourceProductName=Foundation Library
  R OcPu : fl_lib/Electrical/Electrical Elements/Resistor  R=470 Ohm  i_specify=off  i_priority=High  i=0 A  i_nominal_specify=off  i_nominal_unit=A  i_nominal_value=1  v_specify=off  v_priority=High  v=0 V  v_nominal_specify=off  v_nominal_unit=V  v_nominal_value=1
      settings: SourceProductName=Foundation Library
  Sensing : Subsystem
  Supply Rail : ee_lib/Sources/Positive Supply Rail  v0=24 V
      settings: SourceProductName=Electrical  InternalSimscapePortConfiguration="{\"Bottom\":[],\"Left\":[],\"Right\":[{\"id\":\"p\",\"label\":\"\",\"type\":\"foundation.electrical.electrical\"}],\"Top\":[]}"
  Supply Rail Nl : ee_lib/Sources/Positive Supply Rail  v0=24 V
      settings: SourceProductName=Electrical  InternalSimscapePortConfiguration="{\"Bottom\":[],\"Left\":[],\"Right\":[{\"id\":\"p\",\"label\":\"\",\"type\":\"foundation.electrical.electrical\"}],\"Top\":[]}"
  Supply Rail Pl : ee_lib/Sources/Positive Supply Rail  v0=24 V
      settings: SourceProductName=Electrical  InternalSimscapePortConfiguration="{\"Bottom\":[],\"Left\":[],\"Right\":[{\"id\":\"p\",\"label\":\"\",\"type\":\"foundation.electrical.electrical\"}],\"Top\":[]}"
  + : PMIOPort  Side=Right
  - : PMIOPort  Port=2  Side=Right
  +ref : PMIOPort  Port=3  Side=Left
  REV : PMIOPort  Port=4  Side=Left
  connections:
  +/RConn1 -- LegPl/RConn1 -- LegPu/RConn2
  Controlled PWM Voltage/RConn1 -- R OcPl/RConn1 -- R OcPu/LConn1 -- R OcNl/RConn1 -- R OcNu/RConn1
  Supply Rail/RConn1 -- LegNu/RConn1 -- LegPu/RConn1
  Interfacing/RConn1 -- Optocoupler Nl/RConn1 -- Optocoupler Pu/RConn1
  Interfacing/RConn2 -- Optocoupler Nu/RConn1 -- Optocoupler Pl/RConn1
  ERef/LConn1 -- LegNl/RConn2 -- LegPl/RConn2
  -/RConn1 -- LegNl/RConn1 -- LegNu/RConn2
  Optocoupler Nl/LConn1 -- R OcNl/LConn1
  REV/RConn1 -- Interfacing/LConn1
  Optocoupler Pu/RConn2 -- ERef Pu/LConn1
  LegPu/LConn1 -- Optocoupler Pu/LConn2
  LegNl/LConn1 -- Optocoupler Nl/RConn2
  Supply Rail Nl/RConn1 -- Optocoupler Nl/LConn2
  Optocoupler Nu/LConn1 -- R OcNu/LConn1
  R OcPl/LConn1 -- Optocoupler Pl/LConn1
  Supply Rail Pl/RConn1 -- Optocoupler Pl/LConn2
  Controlled PWM Voltage/LConn2 -- ERef PWM nRef/LConn1
  Controlled PWM Voltage/LConn1 -- +ref/RConn1
  Optocoupler Pu/LConn1 -- R OcPu/RConn1
  Optocoupler Nu/RConn2 -- ERef Nu/LConn1
  Controlled PWM Voltage/RConn2 -- ERef PWM REF/LConn1
  Optocoupler Pl/RConn2 -- LegPl/LConn1
  LegNu/LConn1 -- Optocoupler Nu/LConn2

== system Motor_Model/Speed and Current Control/Circuit ==
  V_i : Inport
  V_w : Inport  Port=2
  wRef : Inport  Port=3
  Current Controller : Subsystem
  Speed Controller : Subsystem  Tag=PublishSubsystem
  Vr : PMIOPort  Side=Right
  REV : PMIOPort  Port=2  Side=Right
  wires:
  V_i/1 -> Current Controller/1(V_i)
  V_w/1 -> Speed Controller/1(Y)
  wRef/1 -> Speed Controller/2(R)
  connections:
  Vr/RConn1 -- Current Controller/RConn1
  REV/RConn1 -- Current Controller/RConn2
  Speed Controller/RConn1 -- Current Controller/LConn1

== system Motor_Model/Speed and Current Control/Simulink ==
  V_i : Inport
  V_w : Inport  Port=2
  wRef : Inport  Port=3
  Current Controller : Subsystem
  Speed Controller : Subsystem
  rpm2volts : Gain  Gain=1/296
  Vr : PMIOPort  Side=Right
  REV : PMIOPort  Port=2  Side=Right
  wires:
  Speed Controller/1(V_iref) -> Current Controller/2(V_iref)
  V_i/1 -> Current Controller/1(V_i)
  V_w/1 -> Speed Controller/1(V_w)
  wRef/1 -> rpm2volts/1
  rpm2volts/1 -> Speed Controller/2(V_wref)
  connections:
  Vr/RConn1 -- Current Controller/RConn1
  REV/RConn1 -- Current Controller/RConn2

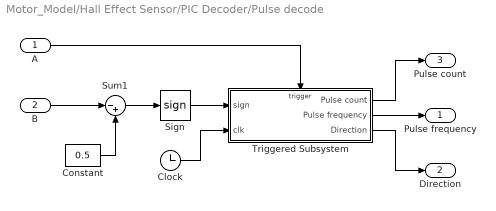
== system Motor_Model/Hall Effect Sensor/PIC Decoder/Pulse decode ==
  A : Inport
  B : Inport  Port=2
  Clock : Clock
  Constant : Constant  Value=0.5
  Sign : Signum
  Sum1 : Sum  Inputs=|-+
  Triggered Subsystem : Subsystem  TreatAsAtomicUnit=on
  Pulse frequency : Outport  VectorParamsAs1DForOutWhenUnconnected=off
  Direction : Outport  Port=2  VectorParamsAs1DForOutWhenUnconnected=off
  Pulse count : Outport  Port=3  VectorParamsAs1DForOutWhenUnconnected=off
  wires:
  Triggered Subsystem/3(Direction) -> Direction/1
  Triggered Subsystem/2(Pulse frequency) -> Pulse frequency/1
  Clock/1 -> Triggered Subsystem/2(clk)
  Triggered Subsystem/1(Pulse count) -> Pulse count/1
  A/1 -> Triggered Subsystem/Trigger
  Sign/1 -> Triggered Subsystem/1(sign)
  B/1 -> Sum1/1
  Sum1/1 -> Sign/1
  Constant/1 -> Sum1/2

== system Motor_Model/Hall Effect Sensor/PIC Decoder/V2SL_1 ==
  ERef3 : fl_lib/Electrical/Electrical Elements/Electrical Reference
      settings: SourceProductName=Foundation Library
  PS-Simulink Converter 2 : nesl_utility/PS-Simulink Converter  PhysicalDomain=network_engine_domain  SubClassName=ps_output  LeftPortType=input  RightPortType=output  PseudoPeriodic=off  Frequencies=[]  Unit=V  AffineConversion=off
      settings: SourceProductName=Utilities
  V2logic : Gain  Gain=0.2
  Voltage Sensor : fl_lib/Electrical/Electrical Sensors/Voltage Sensor
      settings: SourceProductName=Foundation Library
  V : PMIOPort  Side=Left
  SL : Outport  VectorParamsAs1DForOutWhenUnconnected=off
  wires:
  PS-Simulink Converter 2/1 -> V2logic/1
  V2logic/1 -> SL/1
  connections:
  Voltage Sensor/RConn2 -- ERef3/LConn1
  V/RConn1 -- Voltage Sensor/LConn1
  Voltage Sensor/RConn1 -- PS-Simulink Converter 2/LConn1

== system Motor_Model/Hall Effect Sensor/PIC Decoder/V2SL_2 ==
  ERef4 : fl_lib/Electrical/Electrical Elements/Electrical Reference
      settings: SourceProductName=Foundation Library
  PS-Simulink Converter 2 : nesl_utility/PS-Simulink Converter  PhysicalDomain=network_engine_domain  SubClassName=ps_output  LeftPortType=input  RightPortType=output  PseudoPeriodic=off  Frequencies=[]  Unit=V  AffineConversion=off
      settings: SourceProductName=Utilities
  V2logic : Gain  Gain=0.2
  Voltage Sensor : fl_lib/Electrical/Electrical Sensors/Voltage Sensor
      settings: SourceProductName=Foundation Library
  V : PMIOPort  Side=Left
  SL : Outport  VectorParamsAs1DForOutWhenUnconnected=off
  wires:
  V2logic/1 -> SL/1
  PS-Simulink Converter 2/1 -> V2logic/1
  connections:
  Voltage Sensor/RConn1 -- PS-Simulink Converter 2/LConn1
  V/RConn1 -- Voltage Sensor/LConn1
  Voltage Sensor/RConn2 -- ERef4/LConn1

== system Motor_Model/Motor Driver/Abstract/Sensing ==
  ERef12 : fl_lib/Electrical/Electrical Elements/Electrical Reference
      settings: SourceProductName=Foundation Library
  PS-Simulink Converter 2 : nesl_utility/PS-Simulink Converter  PhysicalDomain=network_engine_domain  SubClassName=ps_output  LeftPortType=input  RightPortType=output  PseudoPeriodic=off  Frequencies=[]  Unit=V  AffineConversion=off
      settings: SourceProductName=Utilities
  Voltage Sensor : fl_lib/Electrical/Electrical Sensors/Voltage Sensor
      settings: SourceProductName=Foundation Library
  V : PMIOPort  Side=Left
  Out1 : Outport  VectorParamsAs1DForOutWhenUnconnected=off
  wires:
  PS-Simulink Converter 2/1 -> Out1/1
  connections:
  Voltage Sensor/RConn1 -- PS-Simulink Converter 2/LConn1
  Voltage Sensor/RConn2 -- ERef12/LConn1
  V/RConn1 -- Voltage Sensor/LConn1

== system Motor_Model/Motor Driver/Abstract/Sensing1 ==
  ERef13 : fl_lib/Electrical/Electrical Elements/Electrical Reference
      settings: SourceProductName=Foundation Library
  PS-Simulink Converter 2 : nesl_utility/PS-Simulink Converter  PhysicalDomain=network_engine_domain  SubClassName=ps_output  LeftPortType=input  RightPortType=output  PseudoPeriodic=off  Frequencies=[]  Unit=V  AffineConversion=off
      settings: SourceProductName=Utilities
  Voltage Sensor : fl_lib/Electrical/Electrical Sensors/Voltage Sensor
      settings: SourceProductName=Foundation Library
  V : PMIOPort  Side=Left
  Out1 : Outport  VectorParamsAs1DForOutWhenUnconnected=off
  wires:
  PS-Simulink Converter 2/1 -> Out1/1
  connections:
  V/RConn1 -- Voltage Sensor/LConn1
  Voltage Sensor/RConn2 -- ERef13/LConn1
  Voltage Sensor/RConn1 -- PS-Simulink Converter 2/LConn1
